simulink model "feedforwardPastInputs"  (R2023b)
settings: Solver=VariableStepAuto  StartTime=0.0  StopTime=stopTime  RelTol=1e-3
values from neighbouring files (symbols this model uses):
  D = 0    [mainScript.m]    (also in ode45Practice.m; ode45WithNeuralNetwork.m)
undefined symbols (not defined in the file or in its folder): sampleTime
libraries: cstblocks x2
settings Model: Creator=Bora  LastModifiedBy=Bora

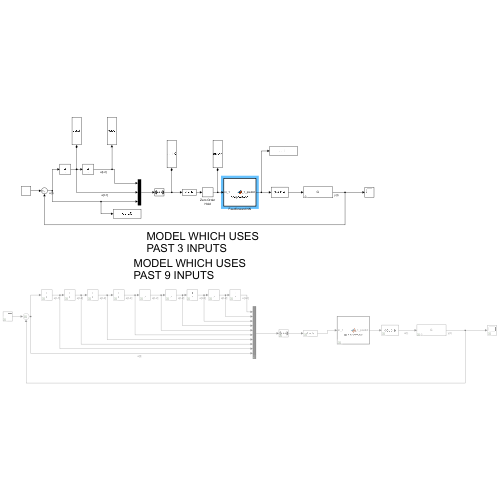
[thumbnail: Simulink's stored preview of the top-level diagram]
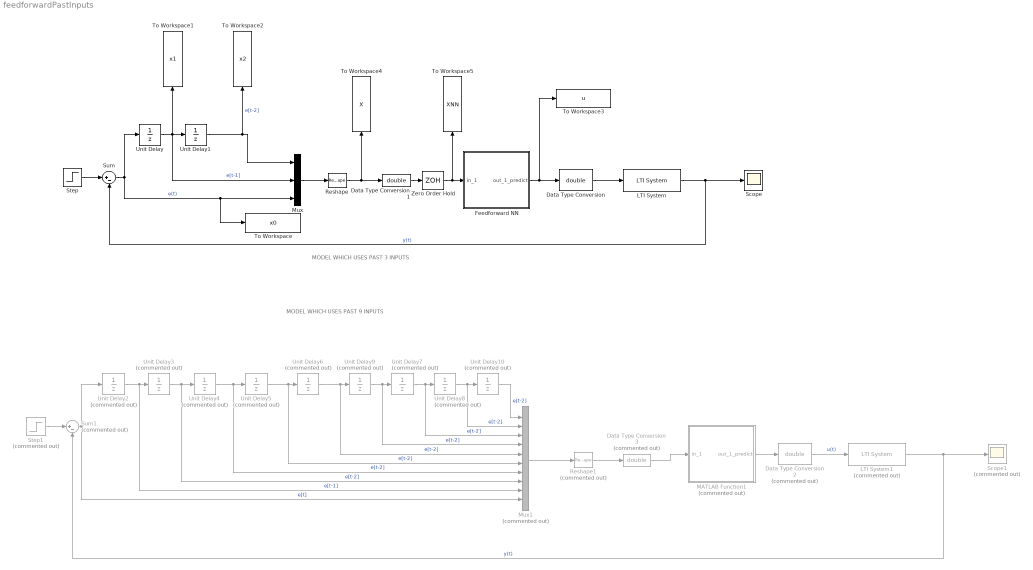
== system feedforwardPastInputs ==
  note: MODEL WHICH USES PAST 9 INPUTS
  note: MODEL WHICH USES PAST 3 INPUTS
  Data Type Conversion : DataTypeConversion  OutDataTypeStr=double  SaturateOnIntegerOverflow=off  RndMeth=Floor
  Data Type Conversion1 : DataTypeConversion  OutDataTypeStr=double  SaturateOnIntegerOverflow=off  RndMeth=Floor
  Data Type Conversion2 : DataTypeConversion  Commented=on  OutDataTypeStr=double  SaturateOnIntegerOverflow=off  RndMeth=Floor
  Data Type Conversion3 : DataTypeConversion  Commented=on  OutDataTypeStr=double  SaturateOnIntegerOverflow=off  RndMeth=Floor
  Feedforward NN : MATLAB Function  TreatAsAtomicUnit=on
  LTI System : cstblocks/LTI System  sys=G  IC=[]  PadeOrder=0
  LTI System1 : cstblocks/LTI System  Commented=on  sys=G  IC=[]  PadeOrder=0
  MATLAB Function1 : MATLAB Function  Commented=on  TreatAsAtomicUnit=on
  Mux : Mux  Inputs=3
  Mux1 : Mux  Commented=on  Inputs=10
  Reshape : Reshape  OutputDimensionality=Row vector (2-D)
  Reshape1 : Reshape  Commented=on  OutputDimensionality=Row vector (2-D)
  Scope : Scope
  Scope1 : Scope  Commented=on
  Step : Step  Time=0  SampleTime=0
  Step1 : Step  Commented=on  Time=0  SampleTime=0
  Sum : Sum  Inputs=|+-
  Sum1 : Sum  Commented=on  Inputs=|+-
  To Workspace : ToWorkspace  VariableName=x0  SaveFormat=Timeseries  SampleTime=sampleTime
  To Workspace1 : ToWorkspace  VariableName=x1  SaveFormat=Timeseries  SampleTime=sampleTime
  To Workspace2 : ToWorkspace  VariableName=x2  SaveFormat=Timeseries  SampleTime=sampleTime
  To Workspace3 : ToWorkspace  VariableName=u  SaveFormat=Timeseries  SampleTime=sampleTime
  To Workspace4 : ToWorkspace  VariableName=X  SaveFormat=Timeseries  SampleTime=sampleTime
  To Workspace5 : ToWorkspace  VariableName=XNN  SaveFormat=Timeseries  SampleTime=sampleTime
  Unit Delay : UnitDelay  SampleTime=sampleTime  HasFrameUpgradeWarning=on
  Unit Delay1 : UnitDelay  SampleTime=sampleTime  HasFrameUpgradeWarning=on
  Unit Delay{2..10} (9 alike) : UnitDelay  Commented=on  SampleTime=sampleTime  HasFrameUpgradeWarning=on
  Zero Order Hold : ZeroOrderHold  SampleTime=sampleTime
  wires:
  Sum/1 -> To Workspace/1, Mux/3, Unit Delay/1  "e(t)"
  Step/1 -> Sum/1
  Unit Delay/1 -> To Workspace1/1, Unit Delay1/1, Mux/2  "e[t-1]"
  Feedforward NN/1(out_1_predict) -> To Workspace3/1, Data Type Conversion/1
  Unit Delay1/1 -> Mux/1, To Workspace2/1  "e[t-2]"
  LTI System/1 -> Scope/1, Sum/2  "y(t)"
  Mux/1 -> Reshape/1
  Reshape/1 -> Data Type Conversion1/1, To Workspace4/1
  Data Type Conversion1/1 -> Zero Order Hold/1
  Data Type Conversion/1 -> LTI System/1
  Reshape1/1 -> Data Type Conversion3/1
  Mux1/1 -> Reshape1/1
  MATLAB Function1/1(out_1_predict) -> Data Type Conversion2/1
  Data Type Conversion2/1 -> LTI System1/1  "u(t)"
  LTI System1/1 -> Scope1/1, Sum1/2  "y(t)"
  Data Type Conversion3/1 -> MATLAB Function1/1(in_1)
  Unit Delay2/1 -> Mux1/9, Unit Delay3/1  "e[t-1]"
  Step1/1 -> Sum1/1
  Sum1/1 -> Mux1/10, Unit Delay2/1  "e[t]"
  Unit Delay3/1 -> Mux1/8, Unit Delay4/1  "e[t-2]"
  Unit Delay4/1 -> Mux1/7, Unit Delay5/1  "e[t-2]"
  Unit Delay5/1 -> Mux1/6, Unit Delay6/1  "e[t-2]"
  Unit Delay6/1 -> Mux1/5, Unit Delay9/1  "e[t-2]"
  Unit Delay9/1 -> Mux1/4, Unit Delay7/1  "e[t-2]"
  Unit Delay7/1 -> Mux1/3, Unit Delay8/1  "e[t-2]"
  Unit Delay8/1 -> Mux1/2, Unit Delay10/1  "e[t-2]"
  Unit Delay10/1 -> Mux1/1  "e[t-2]"
  Zero Order Hold/1 -> To Workspace5/1, Feedforward NN/1(in_1)

== matlab function feedforwardPastInputs/Feedforward NN ==
  data: in_1 input; out_1_predict output
function out_1_predict  = deepNetwork( in_1 )
isSim = coder.target('sfun');
simSupported = false;
useExtrinsic = isSim && ~simSupported;
[out_1_predict] = deep.blocks.internal.deepNetwork({in_1}, {size(in_1)}, {class(in_1)}, coder.const("feedforwardPastInputs/Predict1"), 'C:\Users\Bora\OneDrive - Nexus365\Desktop\4YP MATLAB\RNNnetWithMemory\FeedforwardPastNet.mat', useExtrinsic, false, 128, true, {''}, {});
end

== matlab function feedforwardPastInputs/MATLAB Function1 ==
  data: in_1 input; out_1_predict output
function out_1_predict  = deepNetwork( in_1 )
isSim = coder.target('sfun');
simSupported = false;
useExtrinsic = isSim && ~simSupported;
[out_1_predict] = deep.blocks.internal.deepNetwork({in_1}, {size(in_1)}, {class(in_1)}, coder.const("feedforwardPastInputs/Predict1"), 'C:\Users\Bora\OneDrive - Nexus365\Desktop\4YP MATLAB\RNNnetWithMemory\Past10Inputs.mat', useExtrinsic, false, 128, true, {''}, {});
end
